simulink model "VCU_SW"  (R2020b)
settings: Solver=FixedStepDiscrete  StartTime=0.0  StopTime=inf  FixedStep=1e-2  RelTol=1e-3
PreLoadFcn:
  | RTWConfigurationCB('preloadfcn', bdroot);
InitFcn:
  | loadvar_ttc500
undefined symbols (not defined in the file or in its folder): BrkPedalTypes, CabMovModeTypes, cFuseTempSensAcc_X, cFuseTempSensAcc_Y, cFuseTempSensVal_X, cFuseTempSensVal_Y, cTMSTempSensVal_X, cTMSTempSensVal_Y, cTransferCaseSpeedRatio, diag_state, DoorsPositionTypes, dP_filter_Y, DriverOccClassSystemTypes, ErrorValueTypes, fatal_error_callback, IO_ADC_NO_RANGE, LadderStatusTypes, pAnalogCabRotSensAcc, pAnalogCabRotSensMaxVolt, pAnalogCabRotSensMinVolt, pAnalogCabRotSensRange, pAnalogCabRotSensZeroVolt, pBrkActivePress, pCabTiltSensAcc, pCabTiltSensMaxCur, pCabTiltSensMinCur, pDistanceCorrection, pECANManual_BPNEnable, pECANManual_BPNEnabler_Flag, pFilterSensAccRes, pHDirMaxDiffFrq, pHDirSensHighLvl, pHDirSensLowLvl, pMainGearRatio, pMaxFilterSensRes, pMaxFirstPedalSensValue, pMaxFuseTempSensRes, pMaxPressLoss, pMaxPressSensCurrent, pMaxPressValue, pMaxPressValueHydMotAndPump, pMaxPressValueParkDrain, pMaxSecondPedalSensValue, pMaxTempSensVoltage, pMaxTempValue, pMaxTMSTempSensRes, pMinFilterSensRes, pMinFirstPedalSensValue, pMinFuseTempSensRes, pMinPressLoss, pMinPressSensCurrent, pMinPressValue, pMinSecondPedalSensValue, pMinTempSensVoltage, pMinTempValue, pMinTMSTempSensRes, pMotorRingTeethNum, pPedalSensAccuracyPct, pPedalSensAccuracyVolt, pPressLossTreshhold ... (+20)
libraries: TTlibrary x271, canmsglib x128, simulink x88
(part 12 of 17)

== system VCU_SW/InputLayer/InputNetwork/InputHydCAN/GetHydCAN100msec/Cabine1stLeftHydCylValve ==
  CAN_Unpack_ADDRCL_HYD2 : canmsglib/CAN Unpack  MsgList=(none)  MsgName=ADDRCL_HYD2  MsgIDType=Extended (29-bit identifier)  MsgIdentifier=418315905  MsgLength=8  SignalInfo={ 'ArbitraryAdressStr2', '63', '1', 'LE', 'unsigned', 'Standard', '0', '1', '0', '0', '1'; 'EcuInstanceHyd2', '32', '3', 'LE', 'unsigned', 'Standard', '0', '1', '0', '0', '7'; 'FunctionInstanceHyd2', '35', '5', 'LE', 'unsigned', 'Standard', '0', '1', '0', '0', '31'; 'IdentityNumberDanfossHyd2', '0', '16', 'LE', 'unsigned', 'Standard', '0', '1', '0', '0', '65535'; 'IdentityNumberHyd2', '28', '4', 'LE', 'unsigned', 'Standard', '0', '1', '0', '0', '15'; 'IndustryGroupStr2', '60', '3', 'LE', 'unsigned', 'Standard', '0', '1', '0', '0', '7'; 'ManufacturerCodeStr2', '16', '12', 'LE', 'unsigned', 'Standard', '0', '1', '0', '0', '4095'; 'VehSystemInstanceHyd2', '56', '4', 'LE', 'unsigned', 'Standard', '0', '1', '0', '0', '15'; 'VehicleSystemHyd2', '49', '7', 'LE', 'unsigned', 'Standard', '0', '1', '0', '0', '127' }  IDPort=off  TimestampPort=off  ErrorPort=off  RemotePort=off  LengthPort=off  StatusPort=off  ApplyMinMax=off
      settings: SourceProductBaseCode=ME,XP,VN
  CAN_Unpack_AUX_VLV_EST_HYD2 : canmsglib/CAN Unpack  MsgList=(none)  MsgName=AUX_VLV_EST_HYD2  MsgIDType=Extended (29-bit identifier)  MsgIdentifier=217977217  MsgLength=3  SignalInfo={ 'ExtendPortFlowHyd2', '0', '8', 'LE', 'unsigned', 'Standard', '0', '1', '125', '125', '380'; 'FailSafeModeFlowHyd2', '22', '2', 'LE', 'unsigned', 'Standard', '0', '1', '0', '0', '3'; 'RetractPortFlowHyd2', '8', '8', 'LE', 'unsigned', 'Standard', '0', '1', '125', '125', '380'; 'ValveStateFlowHyd2', '16', '4', 'LE', 'unsigned', 'Standard', '0', '1', '0', '0', '15' }  IDPort=off  TimestampPort=off  ErrorPort=off  RemotePort=off  LengthPort=off  StatusPort=off  ApplyMinMax=off
      settings: SourceProductBaseCode=ME,XP,VN
  DataStoreWrite_ADDRCL_HYD2 : DataStoreWrite  DataStoreName=InputNetworkData  DataStoreElements=InputNetworkData.HydCAN.in_CabineTilt_1LeftHydCyl.arbitaryAdressHyd#InputNetworkData.HydCAN.in_CabineTilt_1LeftHydCyl.ecuInstanceHyd#InputNetworkData.HydCAN.in_CabineTilt_1LeftHydCyl.functionInstanceHyd#InputNetworkData.HydCAN.in_CabineTilt_1LeftHydCyl.identityNumDanfossHyd#InputNetworkData.HydCAN.in_CabineTilt_1LeftHydCyl.identityNumHyd#InputNetworkData.HydCAN.in_CabineTilt_1LeftHydCyl.industryGroupHyd#InputNetworkData.HydCAN.in_CabineTilt_1LeftHydCyl.manufacturerCodeHyd#InputNetworkData.HydCAN.in_CabineTilt_1LeftHydCyl.vehSystemInstanceHyd#InputNetworkData.HydCAN.in_CabineTilt_1LeftHydCyl.vehicleSystemStr
  DataStoreWrite_AUX_VLV_EST_HYD2 : DataStoreWrite  DataStoreName=InputNetworkData  DataStoreElements=InputNetworkData.HydCAN.in_CabineTilt_1LeftHydCyl.extendPortFlowHyd#InputNetworkData.HydCAN.in_CabineTilt_1LeftHydCyl.failSafeModeFlowHyd#InputNetworkData.HydCAN.in_CabineTilt_1LeftHydCyl.retractPortFlowHyd#InputNetworkData.HydCAN.in_CabineTilt_1LeftHydCyl.valveStateFlowHyd
  Terminator : Terminator
  Terminator1 : Terminator
  read_message_ADDRCL_HYD2 : TTlibrary/CAN/read_message_name  channel=IO_CAN_CHANNEL_0  id_format=IO_CAN_EXT_FRAME  get_msg_info=off  message_names=there is no CAN Unpack blocks  message_info=|  id=418315905  ac_mask=536870911  retranslation=off  io_error=on  sample_time=-1
      | Message Name: ADDRCL_HYD2
      |  Message ID Type: Extended (29-bit identifier)
      |  Message ID: 418315905
      settings: SourceProductName=TT control 500 series
  read_message_AUX_VLV_EST_HYD2 : TTlibrary/CAN/read_message_name  channel=IO_CAN_CHANNEL_0  id_format=IO_CAN_EXT_FRAME  get_msg_info=off  message_names=there is no CAN Unpack blocks  message_info=|  id=217977217  ac_mask=536870911  retranslation=off  io_error=on  sample_time=-1
      | Message Name: AUX_VLV_EST_HYD2
      |  Message ID Type: Extended (29-bit identifier)
      |  Message ID: 217977217
      settings: SourceProductName=TT control 500 series
  wires:
  CAN_Unpack_ADDRCL_HYD2/7 -> DataStoreWrite_ADDRCL_HYD2/7
  CAN_Unpack_ADDRCL_HYD2/4 -> DataStoreWrite_ADDRCL_HYD2/4
  read_message_AUX_VLV_EST_HYD2/2 -> Terminator/1  "handler_err_217977217"
  read_message_AUX_VLV_EST_HYD2/1 -> CAN_Unpack_AUX_VLV_EST_HYD2/1  "msg_217977217"
  CAN_Unpack_ADDRCL_HYD2/3 -> DataStoreWrite_ADDRCL_HYD2/3
  CAN_Unpack_ADDRCL_HYD2/6 -> DataStoreWrite_ADDRCL_HYD2/6
  CAN_Unpack_AUX_VLV_EST_HYD2/2 -> DataStoreWrite_AUX_VLV_EST_HYD2/2
  CAN_Unpack_ADDRCL_HYD2/5 -> DataStoreWrite_ADDRCL_HYD2/5
  CAN_Unpack_ADDRCL_HYD2/9 -> DataStoreWrite_ADDRCL_HYD2/9
  CAN_Unpack_ADDRCL_HYD2/8 -> DataStoreWrite_ADDRCL_HYD2/8
  CAN_Unpack_AUX_VLV_EST_HYD2/1 -> DataStoreWrite_AUX_VLV_EST_HYD2/1
  read_message_ADDRCL_HYD2/2 -> Terminator1/1  "handler_err_418315905"
  CAN_Unpack_AUX_VLV_EST_HYD2/3 -> DataStoreWrite_AUX_VLV_EST_HYD2/3
  CAN_Unpack_AUX_VLV_EST_HYD2/4 -> DataStoreWrite_AUX_VLV_EST_HYD2/4
  read_message_ADDRCL_HYD2/1 -> CAN_Unpack_ADDRCL_HYD2/1  "msg_418315905"
  CAN_Unpack_ADDRCL_HYD2/1 -> DataStoreWrite_ADDRCL_HYD2/1
  CAN_Unpack_ADDRCL_HYD2/2 -> DataStoreWrite_ADDRCL_HYD2/2

== system VCU_SW/InputLayer/InputNetwork/InputHydCAN/GetHydCAN100msec/Cabine2ndRightHydCylValve ==
  CAN_Unpack_ADDRCL_HYD3 : canmsglib/CAN Unpack  MsgList=(none)  MsgName=ADDRCL_HYD3  MsgIDType=Extended (29-bit identifier)  MsgIdentifier=418315906  MsgLength=8  SignalInfo={ 'ArbitraryAdressHyd3', '63', '1', 'LE', 'unsigned', 'Standard', '0', '1', '0', '0', '1'; 'EcuInstanceHyd3', '32', '3', 'LE', 'unsigned', 'Standard', '0', '1', '0', '0', '7'; 'FunctionInstanceHyd3', '35', '5', 'LE', 'unsigned', 'Standard', '0', '1', '0', '0', '31'; 'IdentityNumberDanfossHyd3', '0', '16', 'LE', 'unsigned', 'Standard', '0', '1', '0', '0', '65535'; 'IdentityNumberHyd3', '28', '4', 'LE', 'unsigned', 'Standard', '0', '1', '0', '0', '15'; 'IndustryGroupHyd3', '60', '3', 'LE', 'unsigned', 'Standard', '0', '1', '0', '0', '7'; 'ManufacturerCodeHyd3', '16', '12', 'LE', 'unsigned', 'Standard', '0', '1', '0', '0', '4095'; 'VehSystemInstanceHyd3', '56', '4', 'LE', 'unsigned', 'Standard', '0', '1', '0', '0', '15'; 'VehicleSystemHyd3', '49', '7', 'LE', 'unsigned', 'Standard', '0', '1', '0', '0', '127' }  IDPort=off  TimestampPort=off  ErrorPort=off  RemotePort=off  LengthPort=off  StatusPort=off  ApplyMinMax=off
      settings: SourceProductBaseCode=ME,XP,VN
  CAN_Unpack_AUX_VLV_EST_HYD3 : canmsglib/CAN Unpack  MsgList=(none)  MsgName=AUX_VLV_EST_HYD3  MsgIDType=Extended (29-bit identifier)  MsgIdentifier=217977218  MsgLength=3  SignalInfo={ 'ExtendPortFlowHyd3', '0', '8', 'LE', 'unsigned', 'Standard', '0', '1', '125', '125', '225'; 'FailSafeModeFlowHyd3', '22', '2', 'LE', 'unsigned', 'Standard', '0', '1', '0', '0', '3'; 'RetractPortFlowHyd3', '8', '8', 'LE', 'unsigned', 'Standard', '0', '1', '125', '125', '225'; 'ValveStateFlowHyd3', '16', '4', 'LE', 'unsigned', 'Standard', '0', '1', '0', '0', '15' }  IDPort=off  TimestampPort=off  ErrorPort=off  RemotePort=off  LengthPort=off  StatusPort=off  ApplyMinMax=off
      settings: SourceProductBaseCode=ME,XP,VN
  DataStoreWrite_ADDRCL_HYD3 : DataStoreWrite  DataStoreName=InputNetworkData  DataStoreElements=InputNetworkData.HydCAN.in_CabineTilt_2RightHydCyl.arbitaryAdressHyd#InputNetworkData.HydCAN.in_CabineTilt_2RightHydCyl.ecuInstanceHyd#InputNetworkData.HydCAN.in_CabineTilt_2RightHydCyl.functionInstanceHyd#InputNetworkData.HydCAN.in_CabineTilt_2RightHydCyl.identityNumDanfossHyd#InputNetworkData.HydCAN.in_CabineTilt_2RightHydCyl.identityNumHyd#InputNetworkData.HydCAN.in_CabineTilt_2RightHydCyl.industryGroupHyd#InputNetworkData.HydCAN.in_CabineTilt_2RightHydCyl.manufacturerCodeHyd#InputNetworkData.HydCAN.in_CabineTilt_2RightHydCyl.vehSystemInstanceHyd#InputNetworkData.HydCAN.in_CabineTilt_2RightHydCyl.vehicleSystemStr
  DataStoreWrite_AUX_VLV_EST_HYD3 : DataStoreWrite  DataStoreName=InputNetworkData  DataStoreElements=InputNetworkData.HydCAN.in_CabineTilt_2RightHydCyl.extendPortFlowHyd#InputNetworkData.HydCAN.in_CabineTilt_2RightHydCyl.failSafeModeFlowHyd#InputNetworkData.HydCAN.in_CabineTilt_2RightHydCyl.retractPortFlowHyd#InputNetworkData.HydCAN.in_CabineTilt_2RightHydCyl.valveStateFlowHyd
  Terminator : Terminator
  Terminator1 : Terminator
  read_message_ADDRCL_HYD3 : TTlibrary/CAN/read_message_name  channel=IO_CAN_CHANNEL_0  id_format=IO_CAN_EXT_FRAME  get_msg_info=off  message_names=there is no CAN Unpack blocks  message_info=|  id=418315906  ac_mask=536870911  retranslation=off  io_error=on  sample_time=-1
      | Message Name: ADDRCL_HYD3
      |  Message ID Type: Extended (29-bit identifier)
      |  Message ID: 418315906
      settings: SourceProductName=TT control 500 series
  read_message_AUX_VLV_EST_HYD3 : TTlibrary/CAN/read_message_name  channel=IO_CAN_CHANNEL_0  id_format=IO_CAN_EXT_FRAME  get_msg_info=off  message_names=there is no CAN Unpack blocks  message_info=|  id=217977218  ac_mask=536870911  retranslation=off  io_error=on  sample_time=-1
      | Message Name: AUX_VLV_EST_HYD3
      |  Message ID Type: Extended (29-bit identifier)
      |  Message ID: 217977218
      settings: SourceProductName=TT control 500 series
  wires:
  CAN_Unpack_AUX_VLV_EST_HYD3/2 -> DataStoreWrite_AUX_VLV_EST_HYD3/2
  CAN_Unpack_AUX_VLV_EST_HYD3/1 -> DataStoreWrite_AUX_VLV_EST_HYD3/1
  CAN_Unpack_ADDRCL_HYD3/1 -> DataStoreWrite_ADDRCL_HYD3/1
  CAN_Unpack_ADDRCL_HYD3/2 -> DataStoreWrite_ADDRCL_HYD3/2
  read_message_ADDRCL_HYD3/1 -> CAN_Unpack_ADDRCL_HYD3/1  "msg_418315906"
  CAN_Unpack_AUX_VLV_EST_HYD3/4 -> DataStoreWrite_AUX_VLV_EST_HYD3/4
  CAN_Unpack_AUX_VLV_EST_HYD3/3 -> DataStoreWrite_AUX_VLV_EST_HYD3/3
  read_message_ADDRCL_HYD3/2 -> Terminator1/1  "handler_err_418315906"
  CAN_Unpack_ADDRCL_HYD3/8 -> DataStoreWrite_ADDRCL_HYD3/8
  CAN_Unpack_ADDRCL_HYD3/6 -> DataStoreWrite_ADDRCL_HYD3/6
  read_message_AUX_VLV_EST_HYD3/1 -> CAN_Unpack_AUX_VLV_EST_HYD3/1  "msg_217977218"
  read_message_AUX_VLV_EST_HYD3/2 -> Terminator/1  "handler_err_217977218"
  CAN_Unpack_ADDRCL_HYD3/3 -> DataStoreWrite_ADDRCL_HYD3/3
  CAN_Unpack_ADDRCL_HYD3/4 -> DataStoreWrite_ADDRCL_HYD3/4
  CAN_Unpack_ADDRCL_HYD3/5 -> DataStoreWrite_ADDRCL_HYD3/5
  CAN_Unpack_ADDRCL_HYD3/9 -> DataStoreWrite_ADDRCL_HYD3/9
  CAN_Unpack_ADDRCL_HYD3/7 -> DataStoreWrite_ADDRCL_HYD3/7

== system VCU_SW/InputLayer/InputNetwork/InputHydCAN/GetHydCAN100msec/CabineTurningValve ==
  CAN_Unpack_ADDRCL_HYD1 : canmsglib/CAN Unpack  MsgList=(none)  MsgName=ADDRCL_HYD1  MsgIDType=Extended (29-bit identifier)  MsgIdentifier=418316160  MsgLength=8  SignalInfo={ 'ArbitraryAdressHyd1', '63', '1', 'LE', 'unsigned', 'Standard', '0', '1', '0', '0', '1'; 'EcuInstanceHyd1', '32', '3', 'LE', 'unsigned', 'Standard', '0', '1', '0', '0', '7'; 'FunctionInstanceHyd1', '35', '5', 'LE', 'unsigned', 'Standard', '0', '1', '0', '0', '31'; 'IdentityNumberDanfossHyd1', '0', '16', 'LE', 'unsigned', 'Standard', '0', '1', '0', '0', '65535'; 'IdentityNumberHyd1', '28', '4', 'LE', 'unsigned', 'Standard', '0', '1', '0', '0', '15'; 'IndustryGroupHyd1', '60', '3', 'LE', 'unsigned', 'Standard', '0', '1', '0', '0', '7'; 'ManufacturerCodeHyd1', '16', '12', 'LE', 'unsigned', 'Standard', '0', '1', '0', '0', '4095'; 'VehSystemInstanceHyd1', '56', '4', 'LE', 'unsigned', 'Standard', '0', '1', '0', '0', '15'; 'VehicleSystemHyd1', '49', '7', 'LE', 'unsigned', 'Standard', '0', '1', '0', '0', '127' }  IDPort=off  TimestampPort=off  ErrorPort=off  RemotePort=off  LengthPort=off  StatusPort=off  ApplyMinMax=off
      settings: SourceProductBaseCode=ME,XP,VN
  CAN_Unpack_AUX_VLV_EST_HYD1 : canmsglib/CAN Unpack  MsgList=(none)  MsgName=AUX_VLV_EST_HYD1  MsgIDType=Extended (29-bit identifier)  MsgIdentifier=217976960  MsgLength=3  SignalInfo={ 'ExtendPortFlowHyd1', '0', '8', 'LE', 'unsigned', 'Standard', '0', '1', '125', '125', '225'; 'FailSafeModeFlowHyd1', '22', '2', 'LE', 'unsigned', 'Standard', '0', '1', '0', '0', '3'; 'RetractPortFlowHyd1', '8', '8', 'LE', 'unsigned', 'Standard', '0', '1', '125', '125', '225'; 'ValveStateFlowHyd1', '16', '4', 'LE', 'unsigned', 'Standard', '0', '1', '0', '0', '15' }  IDPort=off  TimestampPort=off  ErrorPort=off  RemotePort=off  LengthPort=off  StatusPort=off  ApplyMinMax=off
      settings: SourceProductBaseCode=ME,XP,VN
  DataStoreWrite_ADDRCL_HYD1 : DataStoreWrite  DataStoreName=InputNetworkData  DataStoreElements=InputNetworkData.HydCAN.in_CabineRotationVlv.arbitaryAdressHyd#InputNetworkData.HydCAN.in_CabineRotationVlv.ecuInstanceHyd#InputNetworkData.HydCAN.in_CabineRotationVlv.functionInstanceHyd#InputNetworkData.HydCAN.in_CabineRotationVlv.identityNumDanfossHyd#InputNetworkData.HydCAN.in_CabineRotationVlv.identityNumHyd#InputNetworkData.HydCAN.in_CabineRotationVlv.industryGroupHyd#InputNetworkData.HydCAN.in_CabineRotationVlv.manufacturerCodeHyd#InputNetworkData.HydCAN.in_CabineRotationVlv.vehSystemInstanceHyd#InputNetworkData.HydCAN.in_CabineRotationVlv.vehicleSystemStr
  DataStoreWrite_AUX_VLV_EST_HYD1 : DataStoreWrite  DataStoreName=InputNetworkData  DataStoreElements=InputNetworkData.HydCAN.in_CabineRotationVlv.extendPortFlowHyd#InputNetworkData.HydCAN.in_CabineRotationVlv.failSafeModeFlowHyd#InputNetworkData.HydCAN.in_CabineRotationVlv.retractPortFlowHyd#InputNetworkData.HydCAN.in_CabineRotationVlv.valveStateFlowHyd
  Terminator : Terminator
  Terminator1 : Terminator
  read_message_ADDRCL_HYD1 : TTlibrary/CAN/read_message_name  channel=IO_CAN_CHANNEL_0  id_format=IO_CAN_EXT_FRAME  get_msg_info=off  message_names=there is no CAN Unpack blocks  message_info=|  id=418316160  ac_mask=536870911  retranslation=off  io_error=on  sample_time=-1
      | Message Name: ADDRCL_HYD1
      |  Message ID Type: Extended (29-bit identifier)
      |  Message ID: 418316160
      settings: SourceProductName=TT control 500 series
  read_message_AUX_VLV_EST_HYD1 : TTlibrary/CAN/read_message_name  channel=IO_CAN_CHANNEL_0  id_format=IO_CAN_EXT_FRAME  get_msg_info=off  message_names=there is no CAN Unpack blocks  message_info=|  id=217976960  ac_mask=536870911  retranslation=off  io_error=on  sample_time=-1
      | Message Name: AUX_VLV_EST_HYD1
      |  Message ID Type: Extended (29-bit identifier)
      |  Message ID: 217976960
      settings: SourceProductName=TT control 500 series
  wires:
  CAN_Unpack_ADDRCL_HYD1/9 -> DataStoreWrite_ADDRCL_HYD1/9
  CAN_Unpack_ADDRCL_HYD1/8 -> DataStoreWrite_ADDRCL_HYD1/8
  CAN_Unpack_ADDRCL_HYD1/7 -> DataStoreWrite_ADDRCL_HYD1/7
  CAN_Unpack_ADDRCL_HYD1/6 -> DataStoreWrite_ADDRCL_HYD1/6
  CAN_Unpack_ADDRCL_HYD1/5 -> DataStoreWrite_ADDRCL_HYD1/5
  CAN_Unpack_ADDRCL_HYD1/4 -> DataStoreWrite_ADDRCL_HYD1/4
  CAN_Unpack_ADDRCL_HYD1/3 -> DataStoreWrite_ADDRCL_HYD1/3
  CAN_Unpack_AUX_VLV_EST_HYD1/4 -> DataStoreWrite_AUX_VLV_EST_HYD1/4
  CAN_Unpack_AUX_VLV_EST_HYD1/3 -> DataStoreWrite_AUX_VLV_EST_HYD1/3
  CAN_Unpack_ADDRCL_HYD1/1 -> DataStoreWrite_ADDRCL_HYD1/1
  read_message_ADDRCL_HYD1/1 -> CAN_Unpack_ADDRCL_HYD1/1  "msg_418316160"
  CAN_Unpack_ADDRCL_HYD1/2 -> DataStoreWrite_ADDRCL_HYD1/2
  read_message_ADDRCL_HYD1/2 -> Terminator1/1  "handler_err_418316160"
  read_message_AUX_VLV_EST_HYD1/2 -> Terminator/1  "handler_err_217976960"
  CAN_Unpack_AUX_VLV_EST_HYD1/2 -> DataStoreWrite_AUX_VLV_EST_HYD1/2
  read_message_AUX_VLV_EST_HYD1/1 -> CAN_Unpack_AUX_VLV_EST_HYD1/1  "msg_217976960"
  CAN_Unpack_AUX_VLV_EST_HYD1/1 -> DataStoreWrite_AUX_VLV_EST_HYD1/1

== system VCU_SW/InputLayer/InputNetwork/InputStrCAN/GetStrCAN100msec/BJM1 ==
  CAN_Unpack_Str_BJM1 : canmsglib/CAN Unpack  MsgList=(none)  MsgName=BJM1  MsgIDType=Extended (29-bit identifier)  MsgIdentifier=419288595  MsgLength=8  SignalInfo={ 'J1_X_LeftNegPosSts', '2', '2', 'LE', 'unsigned', 'Standard', '0', '1', '0', '0', '3'; 'J1_X_NeutralPosSts', '0', '2', 'LE', 'unsigned', 'Standard', '0', '1', '0', '0', '3'; 'J1_X_Pos', '6', '10', 'LE', 'unsigned', 'Standard', '0', '0.1', '0', '0', '102'; 'J1_X_RightPosSts', '4', '2', 'LE', 'unsigned', 'Standard', '0', '1', '0', '0', '3'; 'J1_Y_BackNegPosSts', '18', '2', 'LE', 'unsigned', 'Standard', '0', '1', '0', '0', '3'; 'J1_Y_ForwPosSts', '20', '2', 'LE', 'unsigned', 'Standard', '0', '1', '0', '0', '3'; 'J1_Y_NeutralPosSts', '16', '2', 'LE', 'unsigned', 'Standard', '0', '1', '0', '0', '3'; 'J1_Y_Pos', '22', '10', 'LE', 'unsigned', 'Standard', '0', '0.1', '0', '0', '102' }  IDPort=off  TimestampPort=off  ErrorPort=off  RemotePort=off  LengthPort=off  StatusPort=off  ApplyMinMax=off
      settings: SourceProductBaseCode=ME,XP,VN
  Data Store Write : DataStoreWrite  DataStoreName=InputNetworkData  DataStoreElements=InputNetworkData.StrCAN.joystickBckwdPosStt#InputNetworkData.StrCAN.joystickFwdPosStt#InputNetworkData.StrCAN.joystickNeutralPosStt#InputNetworkData.StrCAN.joystickPct
  Function Caller1 : FunctionCaller  FunctionPrototype=rawValue = convUintPinToenumStt(uintValue)  InputArgumentSpecifications=<Enter example>  OutputArgumentSpecifications=<Enter example>
  Function Caller2 : FunctionCaller  FunctionPrototype=rawValue = convUintPinToenumStt(uintValue)  InputArgumentSpecifications=<Enter example>  OutputArgumentSpecifications=<Enter example>
  Function Caller3 : FunctionCaller  FunctionPrototype=rawValue = convUintPinToenumStt(uintValue)  InputArgumentSpecifications=<Enter example>  OutputArgumentSpecifications=<Enter example>
  Terminator{2..6} (5 alike) : Terminator
  read_message_Str_BJM1 : TTlibrary/CAN/read_message_name  channel=IO_CAN_CHANNEL_3  id_format=IO_CAN_EXT_FRAME  get_msg_info=off  message_names=there is no CAN Unpack blocks  message_info=|  id=419288595  ac_mask=536870911  retranslation=off  io_error=on  sample_time=-1
      | Message Name: there is no CAN Unpack blocks
      |  Message ID Type: Extended (29-bit identifier)
      |  Message ID: 419364094
      settings: SourceProductName=TT control 500 series
  wires:
  CAN_Unpack_Str_BJM1/8 -> Data Store Write/4
  CAN_Unpack_Str_BJM1/1 -> Terminator4/1
  read_message_Str_BJM1/2 -> Terminator2/1  "handler_err_419288595"
  CAN_Unpack_Str_BJM1/7 -> Function Caller3/1
  CAN_Unpack_Str_BJM1/4 -> Terminator6/1
  CAN_Unpack_Str_BJM1/2 -> Terminator5/1
  read_message_Str_BJM1/1 -> CAN_Unpack_Str_BJM1/1  "msg_419288595"
  CAN_Unpack_Str_BJM1/3 -> Terminator3/1
  CAN_Unpack_Str_BJM1/5 -> Function Caller2/1
  CAN_Unpack_Str_BJM1/6 -> Function Caller1/1
  Function Caller2/1 -> Data Store Write/1
  Function Caller1/1 -> Data Store Write/2
  Function Caller3/1 -> Data Store Write/3

== system VCU_SW/OutputLayer/OutputInterfaces/DigitalOutput1/SetDO1000msec/Subsystem ==
  In1 : Inport
  Constant : Constant  Value=uint8(1)
  Constant1 : Constant  Value=uint8(2)
  Constant49 : Constant  Value=2  OutDataTypeStr=uint8
  Multiport Switch : MultiPortSwitch  DataPortOrder=Zero-based contiguous  Inputs=2  zeroidx=on
  Relational Operator48 : RelationalOperator  Operator===  OutDataTypeStr=boolean  RndMeth=Simplest
  Out1 : Outport
  wires:
  In1/1 -> Relational Operator48/1
  Constant49/1 -> Relational Operator48/2
  Relational Operator48/1 -> Multiport Switch/1
  Constant/1 -> Multiport Switch/3
  Constant1/1 -> Multiport Switch/2
  Multiport Switch/1 -> Out1/1

== system VCU_SW/OutputLayer/OutputInterfaces/DigitalOutput1/SetDO100msec/Subsystem ==
  In1 : Inport
  Constant : Constant  Value=uint8(1)
  Constant1 : Constant  Value=uint8(2)
  Constant49 : Constant  Value=2  OutDataTypeStr=uint8
  Multiport Switch : MultiPortSwitch  DataPortOrder=Zero-based contiguous  Inputs=2  zeroidx=on
  Relational Operator48 : RelationalOperator  Operator===  OutDataTypeStr=boolean  RndMeth=Simplest
  Out1 : Outport
  wires:
  In1/1 -> Relational Operator48/1
  Constant49/1 -> Relational Operator48/2
  Relational Operator48/1 -> Multiport Switch/1
  Constant/1 -> Multiport Switch/3
  Constant1/1 -> Multiport Switch/2
  Multiport Switch/1 -> Out1/1

== system VCU_SW/OutputLayer/OutputInterfaces/DigitalOutput1/SetDO100msec/Subsystem1 ==
  In1 : Inport
  Constant : Constant  Value=uint8(1)
  Constant1 : Constant  Value=uint8(2)
  Constant49 : Constant  Value=2  OutDataTypeStr=uint8
  Multiport Switch : MultiPortSwitch  DataPortOrder=Zero-based contiguous  Inputs=2  zeroidx=on
  Relational Operator48 : RelationalOperator  Operator===  OutDataTypeStr=boolean  RndMeth=Simplest
  Out1 : Outport
  wires:
  Multiport Switch/1 -> Out1/1
  Constant1/1 -> Multiport Switch/2
  Constant/1 -> Multiport Switch/3
  Relational Operator48/1 -> Multiport Switch/1
  Constant49/1 -> Relational Operator48/2
  In1/1 -> Relational Operator48/1

== system VCU_SW/OutputLayer/OutputInterfaces/DigitalOutput1/SetDO100msec/Subsystem10 ==
  In1 : Inport
  Constant : Constant  Value=uint8(1)
  Constant1 : Constant  Value=uint8(2)
  Constant49 : Constant  Value=2  OutDataTypeStr=uint8
  Multiport Switch : MultiPortSwitch  DataPortOrder=Zero-based contiguous  Inputs=2  zeroidx=on
  Relational Operator48 : RelationalOperator  Operator===  OutDataTypeStr=boolean  RndMeth=Simplest
  Out1 : Outport
  wires:
  In1/1 -> Relational Operator48/1
  Constant49/1 -> Relational Operator48/2
  Relational Operator48/1 -> Multiport Switch/1
  Constant/1 -> Multiport Switch/3
  Constant1/1 -> Multiport Switch/2
  Multiport Switch/1 -> Out1/1

== system VCU_SW/OutputLayer/OutputInterfaces/DigitalOutput1/SetDO100msec/Subsystem11 ==
  In1 : Inport
  Constant : Constant  Value=uint8(1)
  Constant1 : Constant  Value=uint8(2)
  Constant49 : Constant  Value=2  OutDataTypeStr=uint8
  Multiport Switch : MultiPortSwitch  DataPortOrder=Zero-based contiguous  Inputs=2  zeroidx=on
  Relational Operator48 : RelationalOperator  Operator===  OutDataTypeStr=boolean  RndMeth=Simplest
  Out1 : Outport
  wires:
  Multiport Switch/1 -> Out1/1
  Constant1/1 -> Multiport Switch/2
  Constant/1 -> Multiport Switch/3
  Relational Operator48/1 -> Multiport Switch/1
  Constant49/1 -> Relational Operator48/2
  In1/1 -> Relational Operator48/1

== system VCU_SW/OutputLayer/OutputInterfaces/DigitalOutput1/SetDO100msec/Subsystem12 ==
  In1 : Inport
  Constant : Constant  Value=uint8(1)
  Constant1 : Constant  Value=uint8(2)
  Constant49 : Constant  Value=2  OutDataTypeStr=uint8
  Multiport Switch : MultiPortSwitch  DataPortOrder=Zero-based contiguous  Inputs=2  zeroidx=on
  Relational Operator48 : RelationalOperator  Operator===  OutDataTypeStr=boolean  RndMeth=Simplest
  Out1 : Outport
  wires:
  In1/1 -> Relational Operator48/1
  Constant49/1 -> Relational Operator48/2
  Relational Operator48/1 -> Multiport Switch/1
  Constant/1 -> Multiport Switch/3
  Constant1/1 -> Multiport Switch/2
  Multiport Switch/1 -> Out1/1

== system VCU_SW/OutputLayer/OutputInterfaces/DigitalOutput1/SetDO100msec/Subsystem13 ==
  In1 : Inport
  Constant : Constant  Value=uint8(1)
  Constant1 : Constant  Value=uint8(2)
  Constant49 : Constant  Value=2  OutDataTypeStr=uint8
  Multiport Switch : MultiPortSwitch  DataPortOrder=Zero-based contiguous  Inputs=2  zeroidx=on
  Relational Operator48 : RelationalOperator  Operator===  OutDataTypeStr=boolean  RndMeth=Simplest
  Out1 : Outport
  wires:
  Multiport Switch/1 -> Out1/1
  Constant1/1 -> Multiport Switch/2
  Constant/1 -> Multiport Switch/3
  Relational Operator48/1 -> Multiport Switch/1
  Constant49/1 -> Relational Operator48/2
  In1/1 -> Relational Operator48/1

== system VCU_SW/OutputLayer/OutputInterfaces/DigitalOutput1/SetDO100msec/Subsystem14 ==
  In1 : Inport
  Constant : Constant  Value=uint8(1)
  Constant1 : Constant  Value=uint8(2)
  Constant49 : Constant  Value=2  OutDataTypeStr=uint8
  Multiport Switch : MultiPortSwitch  DataPortOrder=Zero-based contiguous  Inputs=2  zeroidx=on
  Relational Operator48 : RelationalOperator  Operator===  OutDataTypeStr=boolean  RndMeth=Simplest
  Out1 : Outport
  wires:
  In1/1 -> Relational Operator48/1
  Constant49/1 -> Relational Operator48/2
  Relational Operator48/1 -> Multiport Switch/1
  Constant/1 -> Multiport Switch/3
  Constant1/1 -> Multiport Switch/2
  Multiport Switch/1 -> Out1/1

== system VCU_SW/OutputLayer/OutputInterfaces/DigitalOutput1/SetDO100msec/Subsystem15 ==
  In1 : Inport
  Constant : Constant  Value=uint8(1)
  Constant1 : Constant  Value=uint8(2)
  Constant49 : Constant  Value=2  OutDataTypeStr=uint8
  Multiport Switch : MultiPortSwitch  DataPortOrder=Zero-based contiguous  Inputs=2  zeroidx=on
  Relational Operator48 : RelationalOperator  Operator===  OutDataTypeStr=boolean  RndMeth=Simplest
  Out1 : Outport
  wires:
  Multiport Switch/1 -> Out1/1
  Constant1/1 -> Multiport Switch/2
  Constant/1 -> Multiport Switch/3
  Relational Operator48/1 -> Multiport Switch/1
  Constant49/1 -> Relational Operator48/2
  In1/1 -> Relational Operator48/1

== system VCU_SW/OutputLayer/OutputInterfaces/DigitalOutput1/SetDO100msec/Subsystem16 ==
  In1 : Inport
  Constant : Constant  Value=uint8(1)
  Constant1 : Constant  Value=uint8(2)
  Constant49 : Constant  Value=2  OutDataTypeStr=uint8
  Multiport Switch : MultiPortSwitch  DataPortOrder=Zero-based contiguous  Inputs=2  zeroidx=on
  Relational Operator48 : RelationalOperator  Operator===  OutDataTypeStr=boolean  RndMeth=Simplest
  Out1 : Outport
  wires:
  In1/1 -> Relational Operator48/1
  Constant49/1 -> Relational Operator48/2
  Relational Operator48/1 -> Multiport Switch/1
  Constant/1 -> Multiport Switch/3
  Constant1/1 -> Multiport Switch/2
  Multiport Switch/1 -> Out1/1

== system VCU_SW/OutputLayer/OutputInterfaces/DigitalOutput1/SetDO100msec/Subsystem17 ==
  In1 : Inport
  Constant : Constant  Value=uint8(1)
  Constant1 : Constant  Value=uint8(2)
  Constant49 : Constant  Value=2  OutDataTypeStr=uint8
  Multiport Switch : MultiPortSwitch  DataPortOrder=Zero-based contiguous  Inputs=2  zeroidx=on
  Relational Operator48 : RelationalOperator  Operator===  OutDataTypeStr=boolean  RndMeth=Simplest
  Out1 : Outport
  wires:
  Multiport Switch/1 -> Out1/1
  Constant1/1 -> Multiport Switch/2
  Constant/1 -> Multiport Switch/3
  Relational Operator48/1 -> Multiport Switch/1
  Constant49/1 -> Relational Operator48/2
  In1/1 -> Relational Operator48/1

== system VCU_SW/OutputLayer/OutputInterfaces/DigitalOutput1/SetDO100msec/Subsystem18 ==
  In1 : Inport
  Constant : Constant  Value=uint8(1)
  Constant1 : Constant  Value=uint8(2)
  Constant49 : Constant  Value=2  OutDataTypeStr=uint8
  Multiport Switch : MultiPortSwitch  DataPortOrder=Zero-based contiguous  Inputs=2  zeroidx=on
  Relational Operator48 : RelationalOperator  Operator===  OutDataTypeStr=boolean  RndMeth=Simplest
  Out1 : Outport
  wires:
  In1/1 -> Relational Operator48/1
  Constant49/1 -> Relational Operator48/2
  Relational Operator48/1 -> Multiport Switch/1
  Constant/1 -> Multiport Switch/3
  Constant1/1 -> Multiport Switch/2
  Multiport Switch/1 -> Out1/1

== system VCU_SW/OutputLayer/OutputInterfaces/DigitalOutput1/SetDO100msec/Subsystem2 ==
  In1 : Inport
  Constant : Constant  Value=uint8(1)
  Constant1 : Constant  Value=uint8(2)
  Constant49 : Constant  Value=2  OutDataTypeStr=uint8
  Multiport Switch : MultiPortSwitch  DataPortOrder=Zero-based contiguous  Inputs=2  zeroidx=on
  Relational Operator48 : RelationalOperator  Operator===  OutDataTypeStr=boolean  RndMeth=Simplest
  Out1 : Outport
  wires:
  In1/1 -> Relational Operator48/1
  Constant49/1 -> Relational Operator48/2
  Relational Operator48/1 -> Multiport Switch/1
  Constant/1 -> Multiport Switch/3
  Constant1/1 -> Multiport Switch/2
  Multiport Switch/1 -> Out1/1

== system VCU_SW/OutputLayer/OutputInterfaces/DigitalOutput1/SetDO100msec/Subsystem3 ==
  In1 : Inport
  Constant : Constant  Value=uint8(1)
  Constant1 : Constant  Value=uint8(2)
  Constant49 : Constant  Value=2  OutDataTypeStr=uint8
  Multiport Switch : MultiPortSwitch  DataPortOrder=Zero-based contiguous  Inputs=2  zeroidx=on
  Relational Operator48 : RelationalOperator  Operator===  OutDataTypeStr=boolean  RndMeth=Simplest
  Out1 : Outport
  wires:
  Multiport Switch/1 -> Out1/1
  Constant1/1 -> Multiport Switch/2
  Constant/1 -> Multiport Switch/3
  Relational Operator48/1 -> Multiport Switch/1
  Constant49/1 -> Relational Operator48/2
  In1/1 -> Relational Operator48/1

== system VCU_SW/OutputLayer/OutputInterfaces/DigitalOutput1/SetDO100msec/Subsystem4 ==
  In1 : Inport
  Constant : Constant  Value=uint8(1)
  Constant1 : Constant  Value=uint8(2)
  Constant49 : Constant  Value=2  OutDataTypeStr=uint8
  Multiport Switch : MultiPortSwitch  DataPortOrder=Zero-based contiguous  Inputs=2  zeroidx=on
  Relational Operator48 : RelationalOperator  Operator===  OutDataTypeStr=boolean  RndMeth=Simplest
  Out1 : Outport
  wires:
  In1/1 -> Relational Operator48/1
  Constant49/1 -> Relational Operator48/2
  Relational Operator48/1 -> Multiport Switch/1
  Constant/1 -> Multiport Switch/3
  Constant1/1 -> Multiport Switch/2
  Multiport Switch/1 -> Out1/1

== system VCU_SW/OutputLayer/OutputInterfaces/DigitalOutput1/SetDO100msec/Subsystem5 ==
  In1 : Inport
  Constant : Constant  Value=uint8(1)
  Constant1 : Constant  Value=uint8(2)
  Constant49 : Constant  Value=2  OutDataTypeStr=uint8
  Multiport Switch : MultiPortSwitch  DataPortOrder=Zero-based contiguous  Inputs=2  zeroidx=on
  Relational Operator48 : RelationalOperator  Operator===  OutDataTypeStr=boolean  RndMeth=Simplest
  Out1 : Outport
  wires:
  Multiport Switch/1 -> Out1/1
  Constant1/1 -> Multiport Switch/2
  Constant/1 -> Multiport Switch/3
  Relational Operator48/1 -> Multiport Switch/1
  Constant49/1 -> Relational Operator48/2
  In1/1 -> Relational Operator48/1

== system VCU_SW/OutputLayer/OutputInterfaces/DigitalOutput1/SetDO100msec/Subsystem6 ==
  In1 : Inport
  Constant : Constant  Value=uint8(1)
  Constant1 : Constant  Value=uint8(2)
  Constant49 : Constant  Value=2  OutDataTypeStr=uint8
  Multiport Switch : MultiPortSwitch  DataPortOrder=Zero-based contiguous  Inputs=2  zeroidx=on
  Relational Operator48 : RelationalOperator  Operator===  OutDataTypeStr=boolean  RndMeth=Simplest
  Out1 : Outport
  wires:
  In1/1 -> Relational Operator48/1
  Constant49/1 -> Relational Operator48/2
  Relational Operator48/1 -> Multiport Switch/1
  Constant/1 -> Multiport Switch/3
  Constant1/1 -> Multiport Switch/2
  Multiport Switch/1 -> Out1/1

== system VCU_SW/OutputLayer/OutputInterfaces/DigitalOutput1/SetDO100msec/Subsystem7 ==
  In1 : Inport
  Constant : Constant  Value=uint8(1)
  Constant1 : Constant  Value=uint8(2)
  Constant49 : Constant  Value=2  OutDataTypeStr=uint8
  Multiport Switch : MultiPortSwitch  DataPortOrder=Zero-based contiguous  Inputs=2  zeroidx=on
  Relational Operator48 : RelationalOperator  Operator===  OutDataTypeStr=boolean  RndMeth=Simplest
  Out1 : Outport
  wires:
  Multiport Switch/1 -> Out1/1
  Constant1/1 -> Multiport Switch/2
  Constant/1 -> Multiport Switch/3
  Relational Operator48/1 -> Multiport Switch/1
  Constant49/1 -> Relational Operator48/2
  In1/1 -> Relational Operator48/1

== system VCU_SW/OutputLayer/OutputInterfaces/DigitalOutput1/SetDO100msec/Subsystem8 ==
  In1 : Inport
  Constant : Constant  Value=uint8(1)
  Constant1 : Constant  Value=uint8(2)
  Constant49 : Constant  Value=2  OutDataTypeStr=uint8
  Multiport Switch : MultiPortSwitch  DataPortOrder=Zero-based contiguous  Inputs=2  zeroidx=on
  Relational Operator48 : RelationalOperator  Operator===  OutDataTypeStr=boolean  RndMeth=Simplest
  Out1 : Outport
  wires:
  In1/1 -> Relational Operator48/1
  Constant49/1 -> Relational Operator48/2
  Relational Operator48/1 -> Multiport Switch/1
  Constant/1 -> Multiport Switch/3
  Constant1/1 -> Multiport Switch/2
  Multiport Switch/1 -> Out1/1

== system VCU_SW/OutputLayer/OutputInterfaces/DigitalOutput1/SetDO100msec/Subsystem9 ==
  In1 : Inport
  Constant : Constant  Value=uint8(1)
  Constant1 : Constant  Value=uint8(2)
  Constant49 : Constant  Value=2  OutDataTypeStr=uint8
  Multiport Switch : MultiPortSwitch  DataPortOrder=Zero-based contiguous  Inputs=2  zeroidx=on
  Relational Operator48 : RelationalOperator  Operator===  OutDataTypeStr=boolean  RndMeth=Simplest
  Out1 : Outport
  wires:
  Multiport Switch/1 -> Out1/1
  Constant1/1 -> Multiport Switch/2
  Constant/1 -> Multiport Switch/3
  Relational Operator48/1 -> Multiport Switch/1
  Constant49/1 -> Relational Operator48/2
  In1/1 -> Relational Operator48/1

== system VCU_SW/OutputLayer/OutputInterfaces/DigitalOutput1/SetDO10msec/Subsystem ==
  In1 : Inport
  Constant : Constant  Value=uint8(1)
  Constant1 : Constant  Value=uint8(2)
  Constant49 : Constant  Value=2  OutDataTypeStr=uint8
  Multiport Switch : MultiPortSwitch  DataPortOrder=Zero-based contiguous  Inputs=2  zeroidx=on
  Relational Operator48 : RelationalOperator  Operator===  OutDataTypeStr=boolean  RndMeth=Simplest
  Out1 : Outport
  wires:
  In1/1 -> Relational Operator48/1
  Constant49/1 -> Relational Operator48/2
  Relational Operator48/1 -> Multiport Switch/1
  Constant/1 -> Multiport Switch/3
  Constant1/1 -> Multiport Switch/2
  Multiport Switch/1 -> Out1/1

== system VCU_SW/OutputLayer/OutputInterfaces/DigitalOutput1/SetDO10msec/Subsystem1 ==
  In1 : Inport
  Constant : Constant  Value=uint8(1)
  Constant1 : Constant  Value=uint8(2)
  Constant49 : Constant  Value=2  OutDataTypeStr=uint8
  Multiport Switch : MultiPortSwitch  DataPortOrder=Zero-based contiguous  Inputs=2  zeroidx=on
  Relational Operator48 : RelationalOperator  Operator===  OutDataTypeStr=boolean  RndMeth=Simplest
  Out1 : Outport
  wires:
  Multiport Switch/1 -> Out1/1
  Constant1/1 -> Multiport Switch/2
  Constant/1 -> Multiport Switch/3
  Relational Operator48/1 -> Multiport Switch/1
  Constant49/1 -> Relational Operator48/2
  In1/1 -> Relational Operator48/1

== system VCU_SW/OutputLayer/OutputInterfaces/DigitalOutput1/SetDO10msec/Subsystem10 ==
  In1 : Inport
  Constant : Constant  Value=uint8(1)
  Constant1 : Constant  Value=uint8(2)
  Constant49 : Constant  Value=2  OutDataTypeStr=uint8
  Multiport Switch : MultiPortSwitch  DataPortOrder=Zero-based contiguous  Inputs=2  zeroidx=on
  Relational Operator48 : RelationalOperator  Operator===  OutDataTypeStr=boolean  RndMeth=Simplest
  Out1 : Outport
  wires:
  Multiport Switch/1 -> Out1/1
  Constant1/1 -> Multiport Switch/2
  Constant/1 -> Multiport Switch/3
  Relational Operator48/1 -> Multiport Switch/1
  Constant49/1 -> Relational Operator48/2
  In1/1 -> Relational Operator48/1

== system VCU_SW/OutputLayer/OutputInterfaces/DigitalOutput1/SetDO10msec/Subsystem11 ==
  In1 : Inport
  Constant : Constant  Value=uint8(1)
  Constant1 : Constant  Value=uint8(2)
  Constant49 : Constant  Value=2  OutDataTypeStr=uint8
  Multiport Switch : MultiPortSwitch  DataPortOrder=Zero-based contiguous  Inputs=2  zeroidx=on
  Relational Operator48 : RelationalOperator  Operator===  OutDataTypeStr=boolean  RndMeth=Simplest
  Out1 : Outport
  wires:
  In1/1 -> Relational Operator48/1
  Constant49/1 -> Relational Operator48/2
  Relational Operator48/1 -> Multiport Switch/1
  Constant/1 -> Multiport Switch/3
  Constant1/1 -> Multiport Switch/2
  Multiport Switch/1 -> Out1/1

== system VCU_SW/OutputLayer/OutputInterfaces/DigitalOutput1/SetDO10msec/Subsystem12 ==
  In1 : Inport
  Constant : Constant  Value=uint8(1)
  Constant1 : Constant  Value=uint8(2)
  Constant49 : Constant  Value=2  OutDataTypeStr=uint8
  Multiport Switch : MultiPortSwitch  DataPortOrder=Zero-based contiguous  Inputs=2  zeroidx=on
  Relational Operator48 : RelationalOperator  Operator===  OutDataTypeStr=boolean  RndMeth=Simplest
  Out1 : Outport
  wires:
  Multiport Switch/1 -> Out1/1
  Constant1/1 -> Multiport Switch/2
  Constant/1 -> Multiport Switch/3
  Relational Operator48/1 -> Multiport Switch/1
  Constant49/1 -> Relational Operator48/2
  In1/1 -> Relational Operator48/1

== system VCU_SW/OutputLayer/OutputInterfaces/DigitalOutput1/SetDO10msec/Subsystem13 ==
  In1 : Inport
  Constant : Constant  Value=uint8(1)
  Constant1 : Constant  Value=uint8(2)
  Constant49 : Constant  Value=2  OutDataTypeStr=uint8
  Multiport Switch : MultiPortSwitch  DataPortOrder=Zero-based contiguous  Inputs=2  zeroidx=on
  Relational Operator48 : RelationalOperator  Operator===  OutDataTypeStr=boolean  RndMeth=Simplest
  Out1 : Outport
  wires:
  In1/1 -> Relational Operator48/1
  Constant49/1 -> Relational Operator48/2
  Relational Operator48/1 -> Multiport Switch/1
  Constant/1 -> Multiport Switch/3
  Constant1/1 -> Multiport Switch/2
  Multiport Switch/1 -> Out1/1

== system VCU_SW/OutputLayer/OutputInterfaces/DigitalOutput1/SetDO10msec/Subsystem14 ==
  In1 : Inport
  Constant : Constant  Value=uint8(1)
  Constant1 : Constant  Value=uint8(2)
  Constant49 : Constant  Value=2  OutDataTypeStr=uint8
  Multiport Switch : MultiPortSwitch  DataPortOrder=Zero-based contiguous  Inputs=2  zeroidx=on
  Relational Operator48 : RelationalOperator  Operator===  OutDataTypeStr=boolean  RndMeth=Simplest
  Out1 : Outport
  wires:
  Multiport Switch/1 -> Out1/1
  Constant1/1 -> Multiport Switch/2
  Constant/1 -> Multiport Switch/3
  Relational Operator48/1 -> Multiport Switch/1
  Constant49/1 -> Relational Operator48/2
  In1/1 -> Relational Operator48/1

== system VCU_SW/OutputLayer/OutputInterfaces/DigitalOutput1/SetDO10msec/Subsystem2 ==
  In1 : Inport
  Constant : Constant  Value=uint8(1)
  Constant1 : Constant  Value=uint8(2)
  Constant49 : Constant  Value=2  OutDataTypeStr=uint8
  Multiport Switch : MultiPortSwitch  DataPortOrder=Zero-based contiguous  Inputs=2  zeroidx=on
  Relational Operator48 : RelationalOperator  Operator===  OutDataTypeStr=boolean  RndMeth=Simplest
  Out1 : Outport
  wires:
  In1/1 -> Relational Operator48/1
  Constant49/1 -> Relational Operator48/2
  Relational Operator48/1 -> Multiport Switch/1
  Constant/1 -> Multiport Switch/3
  Constant1/1 -> Multiport Switch/2
  Multiport Switch/1 -> Out1/1

== system VCU_SW/OutputLayer/OutputInterfaces/DigitalOutput1/SetDO10msec/Subsystem3 ==
  In1 : Inport
  Constant : Constant  Value=uint8(1)
  Constant1 : Constant  Value=uint8(2)
  Constant49 : Constant  Value=2  OutDataTypeStr=uint8
  Multiport Switch : MultiPortSwitch  DataPortOrder=Zero-based contiguous  Inputs=2  zeroidx=on
  Relational Operator48 : RelationalOperator  Operator===  OutDataTypeStr=boolean  RndMeth=Simplest
  Out1 : Outport
  wires:
  Multiport Switch/1 -> Out1/1
  Constant1/1 -> Multiport Switch/2
  Constant/1 -> Multiport Switch/3
  Relational Operator48/1 -> Multiport Switch/1
  Constant49/1 -> Relational Operator48/2
  In1/1 -> Relational Operator48/1

== system VCU_SW/OutputLayer/OutputInterfaces/DigitalOutput1/SetDO10msec/Subsystem4 ==
  In1 : Inport
  Constant : Constant  Value=uint8(1)
  Constant1 : Constant  Value=uint8(2)
  Constant49 : Constant  Value=2  OutDataTypeStr=uint8
  Multiport Switch : MultiPortSwitch  DataPortOrder=Zero-based contiguous  Inputs=2  zeroidx=on
  Relational Operator48 : RelationalOperator  Operator===  OutDataTypeStr=boolean  RndMeth=Simplest
  Out1 : Outport
  wires:
  Multiport Switch/1 -> Out1/1
  Constant1/1 -> Multiport Switch/2
  Constant/1 -> Multiport Switch/3
  Relational Operator48/1 -> Multiport Switch/1
  Constant49/1 -> Relational Operator48/2
  In1/1 -> Relational Operator48/1

== system VCU_SW/OutputLayer/OutputInterfaces/DigitalOutput1/SetDO10msec/Subsystem5 ==
  In1 : Inport
  Constant : Constant  Value=uint8(1)
  Constant1 : Constant  Value=uint8(2)
  Constant49 : Constant  Value=2  OutDataTypeStr=uint8
  Multiport Switch : MultiPortSwitch  DataPortOrder=Zero-based contiguous  Inputs=2  zeroidx=on
  Relational Operator48 : RelationalOperator  Operator===  OutDataTypeStr=boolean  RndMeth=Simplest
  Out1 : Outport
  wires:
  In1/1 -> Relational Operator48/1
  Constant49/1 -> Relational Operator48/2
  Relational Operator48/1 -> Multiport Switch/1
  Constant/1 -> Multiport Switch/3
  Constant1/1 -> Multiport Switch/2
  Multiport Switch/1 -> Out1/1

== system VCU_SW/OutputLayer/OutputInterfaces/DigitalOutput1/SetDO10msec/Subsystem6 ==
  In1 : Inport
  Constant : Constant  Value=uint8(1)
  Constant1 : Constant  Value=uint8(2)
  Constant49 : Constant  Value=2  OutDataTypeStr=uint8
  Multiport Switch : MultiPortSwitch  DataPortOrder=Zero-based contiguous  Inputs=2  zeroidx=on
  Relational Operator48 : RelationalOperator  Operator===  OutDataTypeStr=boolean  RndMeth=Simplest
  Out1 : Outport
  wires:
  Multiport Switch/1 -> Out1/1
  Constant1/1 -> Multiport Switch/2
  Constant/1 -> Multiport Switch/3
  Relational Operator48/1 -> Multiport Switch/1
  Constant49/1 -> Relational Operator48/2
  In1/1 -> Relational Operator48/1

== system VCU_SW/OutputLayer/OutputInterfaces/DigitalOutput1/SetDO10msec/Subsystem7 ==
  In1 : Inport
  Constant : Constant  Value=uint8(1)
  Constant1 : Constant  Value=uint8(2)
  Constant49 : Constant  Value=2  OutDataTypeStr=uint8
  Multiport Switch : MultiPortSwitch  DataPortOrder=Zero-based contiguous  Inputs=2  zeroidx=on
  Relational Operator48 : RelationalOperator  Operator===  OutDataTypeStr=boolean  RndMeth=Simplest
  Out1 : Outport
  wires:
  In1/1 -> Relational Operator48/1
  Constant49/1 -> Relational Operator48/2
  Relational Operator48/1 -> Multiport Switch/1
  Constant/1 -> Multiport Switch/3
  Constant1/1 -> Multiport Switch/2
  Multiport Switch/1 -> Out1/1

== system VCU_SW/OutputLayer/OutputInterfaces/DigitalOutput1/SetDO10msec/Subsystem8 ==
  In1 : Inport
  Constant : Constant  Value=uint8(1)
  Constant1 : Constant  Value=uint8(2)
  Constant49 : Constant  Value=2  OutDataTypeStr=uint8
  Multiport Switch : MultiPortSwitch  DataPortOrder=Zero-based contiguous  Inputs=2  zeroidx=on
  Relational Operator48 : RelationalOperator  Operator===  OutDataTypeStr=boolean  RndMeth=Simplest
  Out1 : Outport
  wires:
  Multiport Switch/1 -> Out1/1
  Constant1/1 -> Multiport Switch/2
  Constant/1 -> Multiport Switch/3
  Relational Operator48/1 -> Multiport Switch/1
  Constant49/1 -> Relational Operator48/2
  In1/1 -> Relational Operator48/1

== system VCU_SW/OutputLayer/OutputInterfaces/DigitalOutput1/SetDO10msec/Subsystem9 ==
  In1 : Inport
  Constant : Constant  Value=uint8(1)
  Constant1 : Constant  Value=uint8(2)
  Constant49 : Constant  Value=2  OutDataTypeStr=uint8
  Multiport Switch : MultiPortSwitch  DataPortOrder=Zero-based contiguous  Inputs=2  zeroidx=on
  Relational Operator48 : RelationalOperator  Operator===  OutDataTypeStr=boolean  RndMeth=Simplest
  Out1 : Outport
  wires:
  In1/1 -> Relational Operator48/1
  Constant49/1 -> Relational Operator48/2
  Relational Operator48/1 -> Multiport Switch/1
  Constant/1 -> Multiport Switch/3
  Constant1/1 -> Multiport Switch/2
  Multiport Switch/1 -> Out1/1

== system VCU_SW/OutputLayer/OutputNetwork/OutputCCAN/SetCCAN1000msec/DD_VCU ==
  CANPack_DD_VCU : canmsglib/CAN Pack  MsgList=(none)  MsgName=DD_VCU  MsgIDType=Extended (29-bit identifier)  MsgIdentifier=419364090  MsgLength=8  Remote=off  ApplyMinMax=off  BusOutput=on  SignalInfo={ 'FuelLevelTank1_vcu', '8', '8', 'LE', 'unsigned', 'Standard', '0', '0.4', '0', '0', '100'; 'WasherFluidLevel_vcu', '0', '8', 'LE', 'unsigned', 'Standard', '0', '0.4', '0', '0', '100' }
      settings: SourceProductBaseCode=ME,XP,VN  DataFormat=manually specified signals
  Data Store Read : DataStoreRead  DataStoreName=OutputNetworkData  DataStoreElements=OutputNetworkData.CCAN.DD_VCU.WasherFluidLevel
  Data Store Read1 : DataStoreRead  DataStoreName=OutputNetworkData  DataStoreElements=OutputNetworkData.CCAN.DD_VCU.FuelLevelTank1
  Terminator1 : Terminator
  transmit_message_dd_vcu : TTlibrary/CAN/transmit_message_name  channel=IO_CAN_CHANNEL_1  id_format=IO_CAN_STD_FRAME  retranslation=off  io_error=on  sample_time=-1
      settings: SourceProductName=TT control 500 series
  wires:
  transmit_message_dd_vcu/1 -> Terminator1/1  "error_tx_transmit_message_dd_vcu"
  CANPack_DD_VCU/1 -> transmit_message_dd_vcu/1
  Data Store Read/1 -> CANPack_DD_VCU/2
  Data Store Read1/1 -> CANPack_DD_VCU/1

== system VCU_SW/OutputLayer/OutputNetwork/OutputCCAN/SetCCAN1000msec/DLCC1 ==
  CANPack_DLCC1 : canmsglib/CAN Pack  MsgList=(none)  MsgName=DLCC1  MsgIDType=Extended (29-bit identifier)  MsgIdentifier=419235834  MsgLength=8  Remote=off  ApplyMinMax=off  BusOutput=on  SignalInfo={ 'EngAirFilterRestrictLampCmd', '24', '2', 'LE', 'unsigned', 'Standard', '0', '1', '0', '0', '3'; 'Engine_Amber_Warning_Lamp_Comm', '2', '2', 'LE', 'unsigned', 'Standard', '0', '1', '0', '0', '3'; 'Engine_Coolant_LevLowLampComm', '16', '2', 'LE', 'unsigned', 'Standard', '0', '1', '0', '0', '3'; 'Engine_Coolant_TempHighLampComm', '14', '2', 'LE', 'unsigned', 'Standard', '0', '1', '0', '0', '3'; 'Engine_Oil_PressureLowLamp_Comm', '12', '2', 'LE', 'unsigned', 'Standard', '0', '1', '0', '0', '3'; 'Engine_Protect_Lamp_Command', '0', '2', 'LE', 'unsigned', 'Standard', '0', '1', '0', '0', '3'; 'Engine_RedStop_Lamp_Comm', '4', '2', 'LE', 'unsigned', 'Standard', '0', '1', '0', '0', '3' }
      settings: SourceProductBaseCode=ME,XP,VN  DataFormat=manually specified signals
  Data Store Read1 : DataStoreRead  DataStoreName=OutputNetworkData  DataStoreElements=OutputNetworkData.CCAN.DLCC1.EngAirFilterRestrictLampCmd#OutputNetworkData.CCAN.DLCC1.Engine_Amber_Warning_Lamp_Comm#OutputNetworkData.CCAN.DLCC1.Engine_Coolant_LevLowLampComm#OutputNetworkData.CCAN.DLCC1.Engine_Coolant_TempHighLampComm#OutputNetworkData.CCAN.DLCC1.Engine_Oil_PressureLowLamp_Comm#OutputNetworkData.CCAN.DLCC1.Engine_Protect_Lamp_Command#OutputNetworkData.CCAN.DLCC1.Engine_RedStop_Lamp_Comm
  Terminator1 : Terminator
  transmit_message_dlcc1 : TTlibrary/CAN/transmit_message_name  channel=IO_CAN_CHANNEL_1  id_format=IO_CAN_STD_FRAME  retranslation=off  io_error=on  sample_time=-1
      settings: SourceProductName=TT control 500 series
  wires:
  Data Store Read1/7 -> CANPack_DLCC1/7
  Data Store Read1/6 -> CANPack_DLCC1/6
  Data Store Read1/5 -> CANPack_DLCC1/5
  Data Store Read1/4 -> CANPack_DLCC1/4
  Data Store Read1/3 -> CANPack_DLCC1/3
  Data Store Read1/2 -> CANPack_DLCC1/2
  CANPack_DLCC1/1 -> transmit_message_dlcc1/1
  Data Store Read1/1 -> CANPack_DLCC1/1
  transmit_message_dlcc1/1 -> Terminator1/1  "error_tx_transmit_message_dlcc1"

== system VCU_SW/OutputLayer/OutputNetwork/OutputCCAN/SetCCAN1000msec/DLCC2  ==
  CANPack_DLCC2 : canmsglib/CAN Pack  MsgList=(none)  MsgName=DLCC2  MsgIDType=Extended (29-bit identifier)  MsgIdentifier=419235578  MsgLength=8  Remote=off  ApplyMinMax=off  BusOutput=on  SignalInfo={ 'LowFuelLvl', '2', '2', 'LE', 'unsigned', 'Standard', '0', '1', '0', '0', '3'; 'Vehicle_Batt_ChargingLampCom', '8', '2', 'LE', 'unsigned', 'Standard', '0', '1', '0', '0', '3'; 'Vehicle_Batt_VoltageLowLampCom', '0', '2', 'LE', 'unsigned', 'Standard', '0', '1', '0', '0', '3' }
      settings: SourceProductBaseCode=ME,XP,VN  DataFormat=manually specified signals
  Data Store Read1 : DataStoreRead  DataStoreName=OutputNetworkData  DataStoreElements=OutputNetworkData.CCAN.DLCC2.LowFuelLvl#OutputNetworkData.CCAN.DLCC2.Vehicle_Batt_ChargingLampCom#OutputNetworkData.CCAN.DLCC2.Vehicle_Batt_VoltageLowLampCom
  Terminator1 : Terminator
  transmit_message_dlcc2 : TTlibrary/CAN/transmit_message_name  channel=IO_CAN_CHANNEL_1  id_format=IO_CAN_STD_FRAME  retranslation=off  io_error=on  sample_time=-1
      settings: SourceProductName=TT control 500 series
  wires:
  Data Store Read1/2 -> CANPack_DLCC2/2
  CANPack_DLCC2/1 -> transmit_message_dlcc2/1
  Data Store Read1/1 -> CANPack_DLCC2/1
  transmit_message_dlcc2/1 -> Terminator1/1  "error_tx_transmit_message_dlcc2"
  Data Store Read1/3 -> CANPack_DLCC2/3

== system VCU_SW/OutputLayer/OutputNetwork/OutputCCAN/SetCCAN1000msec/ET1  ==
  CANPack_ET1 : canmsglib/CAN Pack  MsgList=(none)  MsgName=ET1  MsgIDType=Extended (29-bit identifier)  MsgIdentifier=419360506  MsgLength=8  Remote=off  ApplyMinMax=off  BusOutput=on  SignalInfo={ 'Engine_Coolant_Temperature', '0', '8', 'LE', 'unsigned', 'Standard', '0', '1', '-40', '-40', '210'; 'Engine_Fuel_Temperature', '8', '8', 'LE', 'unsigned', 'Standard', '0', '1', '-40', '-40', '210' }
      settings: SourceProductBaseCode=ME,XP,VN  DataFormat=manually specified signals
  Data Store Read1 : DataStoreRead  DataStoreName=OutputNetworkData  DataStoreElements=OutputNetworkData.CCAN.ET1.Engine_Coolant_Temperature#OutputNetworkData.CCAN.ET1.Engine_Fuel_Temperature
  Terminator1 : Terminator
  transmit_message_et1 : TTlibrary/CAN/transmit_message_name  channel=IO_CAN_CHANNEL_1  id_format=IO_CAN_STD_FRAME  retranslation=off  io_error=on  sample_time=-1
      settings: SourceProductName=TT control 500 series
  wires:
  Data Store Read1/2 -> CANPack_ET1/2
  CANPack_ET1/1 -> transmit_message_et1/1
  Data Store Read1/1 -> CANPack_ET1/1
  transmit_message_et1/1 -> Terminator1/1  "error_tx_transmit_message_et1"
